simulink model "ahm_model_no_actuators"  (R2024b)
settings: Solver=FixedStepAuto  StartTime=0.0  StopTime=TMax  FixedStep=DT  RelTol=1e-3
settings Model: Creator=mcdevin  LastModifiedBy=mcdevin

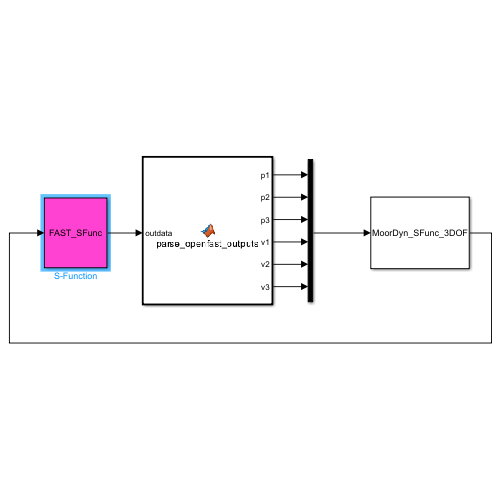
[thumbnail: Simulink's stored preview of the top-level diagram]
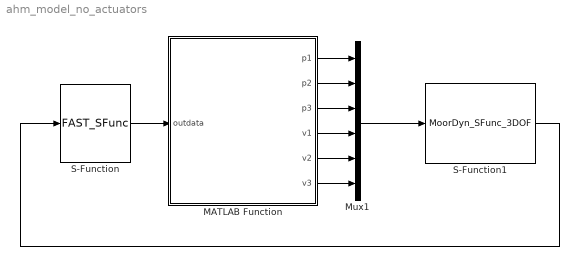
== system ahm_model_no_actuators ==
  MATLAB Function : MATLAB Function  TreatAsAtomicUnit=on
  Mux1 : Mux  Inputs=6
  S-Function : S-Function  FunctionName=FAST_SFunc  Parameters=FAST_InputFileName, TMax, 0  SFunctionDeploymentMode=off  EnableBusSupport=off
  S-Function1 : S-Function  FunctionName=MoorDyn_SFunc_3DOF  Parameters=MD_InputFileName, DT, TMax  SFunctionDeploymentMode=off  EnableBusSupport=off
  wires:
  S-Function1/1 -> S-Function/1
  Mux1/1 -> S-Function1/1
  MATLAB Function/1(p1) -> Mux1/1
  MATLAB Function/2(p2) -> Mux1/2
  MATLAB Function/3(p3) -> Mux1/3
  MATLAB Function/4(v1) -> Mux1/4
  MATLAB Function/5(v2) -> Mux1/5
  MATLAB Function/6(v3) -> Mux1/6
  S-Function/1 -> MATLAB Function/1(outdata)

== matlab function ahm_model_no_actuators/MATLAB Function ==
  data: outdata input; p1 output; p2 output; p3 output; v1 output; v2 output; v3 output
function [p1, p2, p3, v1, v2, v3] = parse_openfast_outputs(outdata)

p1 = outdata(2:4);
p2 = outdata(5:7);
p3 = outdata(8:10);
v1 = outdata(11:13);
v2 = outdata(14:16);
v3 = outdata(17:19);

end
